simulink model "Final_System_Model_V2"  (R2018a)
settings: Solver=VariableStepAuto  StartTime=0  StopTime=inf  RelTol=1e-3
PreLoadFcn:
  | Ts_Power=1e-6;
  | Ts_Control=100e-6;
undefined symbols (not defined in the file): DiscIntNeverNeededParam, FC, FuelCellLoadFcn, gcbh, Ion, Lithium, sigbuilder_block, sps_rtmsupport
libraries: powerlib x20, simulink x10, fl_lib x8, nesl_utility x6, powerlib_meascontrol x5, electricdrivelib x1, spsFuelCellModel x1, re_lib x1
(part 3 of 4)

== system Final_System_Model_V2/180KW Fuel Cell Stack/Load ==
  note: This Block models the Load Profile as dictated by the ship Resistance in the River Nile
  Signal : Inport
  Bus Selector : BusSelector  OutputSignals=Cell Output Voltage (V),Number Of Cells
  Current from Load profile of one day : Subsystem  Tag=STV Subsys  LoadFcn=sigbuilder_block('load');  StartFcn=sigbuilder_block('start');  StopFcn=sigbuilder_block('stop');  ClipboardFcn=sigbuilder_block('clipboard');  mask(Sigbuilder block){tuvar=[0:10]}
      mask help: Simulink:masks:SigbuilderBlock_MD
      mask init:
      | if ~strcmp(get_param(bdroot(gcbh),'SimulationStatus'),'stopped') tuvar = sigbuilder_block('maskInit'); end
      settings: CopyFcn=sigbuilder_block('copy');  DeleteFcn=sigbuilder_block('delete');  ModelCloseFcn=sigbuilder_block('modelClose');  PreSaveFcn=sigbuilder_block('preSave');  PauseFcn=sigbuilder_block('pause');  ContinueFcn=sigbuilder_block('continue');  NameChangeFcn=sigbuilder_block('namechange');  OpenFcn=sigbuilder_block('open',[403.5 117 550.5 359.25 ]);  CloseFcn=sigbuilder_block('close');
      mask Display: plot(0, 0, 100, 100,[2, 2, 32, 32, 2], [68, 8, 8, 68, 68],[32, 2], [38, 38], [32, 19, 2],[53, 60, 44], [32, 17, 17, 2],[16, 16, 31, 31]);txt = getActiveGroup(gcbh);text(2, 100, txt,'verticalAlignment', 'top');
  Product : Product
  Terminator : Terminator
  Terminator1 : Terminator
  Total Output Voltage (V) : Outport
  wires:
  Signal/1 -> Bus Selector/1
  Bus Selector/1 -> Product/1  "<Cell Output Voltage (V)>"
  Product/1 -> Total Output Voltage (V)/1  "Total Output Voltage (V)"
  Current from Load profile of one day/2(Signal 2) -> Terminator1/1  "Current from Load profile (Alex to Aswan)"
  Bus Selector/2 -> Product/2  "<Number Of Cells>"
  Current from Load profile of one day/1(Signal 1) -> Terminator/1  "Current from Load profile (Alex to Aswan)"

== system Final_System_Model_V2/DC-DC converter/Subsystem ==
  duty cycle : Inport
  I in : Inport  Port=2
  V in : Inport  Port=3
  Constant : Constant
  I out : Product  Inputs=*/
  Multiply : Product
  Multiply1 : Product
  Subtract : Sum  Inputs=+-
  V out : Product  Inputs=*/
  efficiency : Gain  Gain=0.98
  efficiency1 : Gain  Gain=0.98
  I o : Outport
  V o : Outport  Port=2
  wires:
  Subtract/1 -> Multiply/1, V out/2
  efficiency/1 -> Multiply/2
  Multiply/1 -> I out/1
  Constant/1 -> Subtract/1
  duty cycle/1 -> Subtract/2, I out/2, Multiply1/2
  Multiply1/1 -> V out/1
  efficiency1/1 -> Multiply1/1
  I in/1 -> efficiency/1
  V out/1 -> V o/1
  I out/1 -> I o/1
  V in/1 -> efficiency1/1

== system Final_System_Model_V2/DC-DC converter/duty cycle ==
  V in : Inport
  V req : Inport  Port=2
  Add : Sum
  Constant : Constant
  Divide : Product  Inputs=*/
  Gain : Gain  Gain=0.98
  Subtract : Sum  Inputs=+-
  tag scope: duty_cycle=global
  wires:
  Subtract/1 -> [duty_cycle]
  V req/1 -> Add/2
  V in/1 -> Gain/1
  Constant/1 -> Subtract/1
  Add/1 -> Divide/2
  Gain/1 -> Divide/1, Add/1
  Divide/1 -> Subtract/2

== system Final_System_Model_V2/Electrolyzer Stack/electrolyser stack ==
  In1 : Inport
  In2 : Inport  Port=2
  Gain : Gain  Gain=2
  Multiply : Product
  Multiply1 : Product
  area in cm^2 : Constant  Value=428
  electrolyser cell : Subsystem
  number of cells : Constant  Value=212
  voltage : Scope
  Out1 : Outport
  Out3 : Outport  Port=2
  wires:
  area in cm^2/1 -> electrolyser cell/3(In3)
  Multiply/1 -> Out1/1
  number of cells/1 -> Multiply1/1, Multiply/1
  electrolyser cell/1(Out1) -> voltage/1, Multiply/2
  In1/1 -> electrolyser cell/1(In1)
  In2/1 -> electrolyser cell/2(In2)
  electrolyser cell/2(Out2) -> Gain/1
  Gain/1 -> Multiply1/2
  Multiply1/1 -> Out3/1

== system Final_System_Model_V2/OLD Version Models/Electrolyser ==
  In1 : Inport
  Electrolyser : Subsystem
  Kg/h : Outport
  wires:
  Electrolyser/1(Kg/h) -> Kg/h/1
  In1/1 -> Electrolyser/1(Current (A))

== system Final_System_Model_V2/OLD Version Models/Fuel Cell ==
  "Hydrogen Flow Rate (kg/s) " : Inport
  Fuel Mass Flow Rate (kg/s) To Current (A) : Subsystem
  Gain : Gain  Gain=0.001
  Number of Cells : Constant  Value=208
  Product : Product
  Output Current : Outport
  Output Voltage (V) : Outport  Port=2
  Output Power (KW) : Outport  Port=3
  wires:
  Number of Cells/1 -> Fuel Mass Flow Rate (kg/s) To Current (A)/2(Number Of Cells)
  "Hydrogen Flow Rate (kg/s) "/1 -> Fuel Mass Flow Rate (kg/s) To Current (A)/1(Hydrogen Flow Rate (kg/s))
  Fuel Mass Flow Rate (kg/s) To Current (A)/1(Current (A)) -> Product/1, Output Current/1
  Fuel Mass Flow Rate (kg/s) To Current (A)/2(Output Voltage (V)) -> Product/2, Output Voltage (V)/1
  Product/1 -> Gain/1
  Gain/1 -> Output Power (KW)/1

== system Final_System_Model_V2/OLD Version Models/Fuel Cell Stack ==
  FuelFr : Inport
  AirFr : Constant  Value=FC.Uf_O2
  Controlled Voltage Source1 : powerlib/Electrical Sources/Controlled Voltage Source  Initialize=on  Source_Type=AC  Amplitude=0  Phase=0  Frequency=0  Measurements=None
  Current Measurement1 : powerlib/Measurements/Current Measurement  PhasorSimulation=off  OutputType=Complex  PSBequivalent=0
  Diode1 : powerlib/Power Electronics/Diode  Ron=FC.Rohm  Lon=0  Vf=0  IC=0  UseSnubber=off  Rs=1e4  Cs=inf  Measurements=off
  Gain1 : Gain  Gain=0.01
  Gain3 : Gain  Gain=0.01
  Model : Subsystem  BlockChoice=Discrete/Detailed
      settings: AttributesFormatString=%<BlockChoice>  TemplateBlock=spsFuelCellModel/Fuel Cell model  MemberBlocks=Continuous/Detailed,Continuous/Simplified,Discrete/Detailed,Discrete/Simplified
  PAir : Constant  Value=FC.PAir
  Pfuel : Constant  Value=FC.Pf
  T : Constant  Value=FC.Tnom
  x_H2 : Constant  Value=FC.x*100
  y_O2 : Constant  Value=FC.y*100
  + : PMIOPort  Tag=PMCPort  Side=Right
  - : PMIOPort  Tag=PMCPort  Port=2  Side=Right
  m : Outport
  wires:
  PAir/1 -> Model/8(PAir)
  Pfuel/1 -> Model/7(Pf)
  T/1 -> Model/2(Op Temp)
  Model/1(Voltage) -> Controlled Voltage Source1/1
  Current Measurement1/1 -> Model/1(Current)
  Model/2(m) -> m/1
  FuelFr/1 -> Model/3(H2)
  x_H2/1 -> Gain1/1
  AirFr/1 -> Model/5(Air)
  y_O2/1 -> Gain3/1
  Gain1/1 -> Model/4(x_H2)
  Gain3/1 -> Model/6(y_O2)
  connections:
  Current Measurement1/LConn1 -- Controlled Voltage Source1/RConn1
  Current Measurement1/RConn1 -- Diode1/LConn1
  -/RConn1 -- Controlled Voltage Source1/LConn1
  Diode1/RConn1 -- +/RConn1

== system Final_System_Model_V2/OLD Version Models/Subsystem ==
  duty_cycle : Inport
  I in : Inport  Port=2
  V in : Inport  Port=3
  Constant : Constant
  I out : Product  Inputs=*/
  Multiply : Product
  Multiply1 : Product
  Subtract : Sum  Inputs=+-
  V out : Product  Inputs=*/
  efficiency : Gain  Gain=0.98
  efficiency1 : Gain  Gain=0.98
  I o : Outport
  V o : Outport  Port=2
  wires:
  Subtract/1 -> Multiply/1, V out/2
  efficiency/1 -> Multiply/2
  Multiply/1 -> I out/1
  Constant/1 -> Subtract/1
  duty_cycle/1 -> Subtract/2, I out/2, Multiply1/2
  Multiply1/1 -> V out/1
  efficiency1/1 -> Multiply1/1
  I in/1 -> efficiency/1
  V out/1 -> V o/1
  I out/1 -> I o/1
  V in/1 -> efficiency1/1

== system Final_System_Model_V2/OLD Version Models/TANK ==
  Input Hydrogen From Electrolyzer (Kg/s) : Inport
  Clock : Clock
  Constant : Constant  Value=700
  Divide : Product  Inputs=*/
  If : If  IfExpression=u1 >= 70.91e6  ShowElse=off
  If Action Subsystem : Subsystem  TreatAsAtomicUnit=on
  J/kgK : Constant  Value=4124.3
  Product : Product
  Product1 : Product  Inputs=3
  Saturation : Saturate  UpperLimit=700  LowerLimit=1
  Simulink-PS Converter : nesl_utility/Simulink-PS Converter  PhysicalDomain=network_engine_domain  SubClassName=ps_input  LeftPortType=input  RightPortType=output  PseudoPeriodic=off  Frequencies=[]  NoiseDistribution=none  NoiseParameters=[]  Unit=Pa  AffineConversion=off  FilteringAndDerivatives=provide  SimscapeFilterOrder=1  InputFilterTimeConstant=0.001  UdotUserProvided=0
  Simulink-PS Converter1 : nesl_utility/Simulink-PS Converter  PhysicalDomain=network_engine_domain  SubClassName=ps_input  LeftPortType=input  RightPortType=output  PseudoPeriodic=off  Frequencies=[]  NoiseDistribution=none  NoiseParameters=[]  Unit=K  AffineConversion=off  FilteringAndDerivatives=provide  SimscapeFilterOrder=1  InputFilterTimeConstant=0.001  UdotUserProvided=0
  Tank Volume (m^3) : Constant
  Temp (K) : Constant  Value=353.15
  Pressure (Pa) : PMIOPort  Side=Right
  Temp1 (K) : PMIOPort  Port=2  Side=Right
  wires:
  Product1/1 -> Divide/1
  Temp (K)/1 -> Simulink-PS Converter1/1, Product1/3
  Input Hydrogen From Electrolyzer (Kg/s)/1 -> Product/1
  Tank Volume (m^3)/1 -> Divide/2
  If Action Subsystem/1(Out1) -> Saturation/1
  Clock/1 -> Product/2
  If/1 -> If Action Subsystem/Action
  Product/1 -> Product1/1  "Mass in Tank (Kg)"
  Divide/1 -> If/1  "Pressure (Pa)"
  Constant/1 -> If Action Subsystem/1(In1)
  J/kgK/1 -> Product1/2
  Saturation/1 -> Simulink-PS Converter/1
  connections:
  Pressure (Pa)/RConn1 -- Simulink-PS Converter/RConn1
  Temp1 (K)/RConn1 -- Simulink-PS Converter1/RConn1

== system Final_System_Model_V2/OLD Version Models/converter ==
  In1 : Inport
  In2 : Inport  Port=2
  Divide : Product  Inputs=*/
  Gain : Gain  Gain=0.98
  Out1 : Outport
  wires:
  Gain/1 -> Divide/2
  In1/1 -> Divide/1
  Divide/1 -> Out1/1
  In2/1 -> Gain/1

== system Final_System_Model_V2/Solar Panel + Solar Charge Controller/PV Insert inputs here ==
  V_PV : Inport
  PV num : Inport  Port=2
  I_sc : Constant  Value=6.39
  Ns_cells : Constant  Value=96
  Product : Product
  Rp : Constant  Value=884.5
  Scope : Scope
  Subsystem : Subsystem
  Temp : Step  Time=5  Before=25  After=25  SampleTime=0
  V_oc : Constant  Value=68.2
  radiation ratio : Step  Before=1  SampleTime=0
  I_PV : Outport
  wires:
  Subsystem/1(I_PV) -> Scope/1, Product/2  "I_PV(A)"
  Temp/1 -> Subsystem/3(T_o)  "Temperature(c)"
  radiation ratio/1 -> Subsystem/2(insolation)  "Radiation ratio"
  Rp/1 -> Subsystem/4(Rp)  "Rp(ohm)"
  V_PV/1 -> Subsystem/1(V_PV)  "V_PV (volt)"
  Product/1 -> I_PV/1
  PV num/1 -> Product/1
  I_sc/1 -> Subsystem/5(I_sc)
  Ns_cells/1 -> Subsystem/6(Ns cells)
  V_oc/1 -> Subsystem/7(V_oc)

== system Final_System_Model_V2/Solar Panel + Solar Charge Controller/Solar Charge Controller ==
  note: 5 kHz - 500V
      | Boost Converter
  m : Inport
  Bus Selector : BusSelector  OutputSignals=V_PV,I_PV
  C1 : powerlib/Elements/Series RLC Branch  LConnTagsString=__new0  RConnTagsString=__new0  BranchType=C  Resistance=1.0  Inductance=1.0  SetiL0=off  InitialCurrent=0  Capacitance=12000e-06  Setx0=off  InitialVoltage=0  Measurements=None
  C2 : powerlib/Elements/Series RLC Branch  LConnTagsString=__new0  RConnTagsString=__new0  BranchType=C  Resistance=1.0  Inductance=1.0  SetiL0=off  InitialCurrent=0  Capacitance=12000e-06  Setx0=off  InitialVoltage=0  Measurements=None
  C3 : powerlib/Elements/Series RLC Branch  LConnTagsString=__new0  RConnTagsString=__new0  BranchType=C  Resistance=1.0  Inductance=1.0  SetiL0=off  InitialCurrent=0  Capacitance=100e-6  Setx0=off  InitialVoltage=0  Measurements=Branch voltage
  Deblock Converters : Step  Time=.05  SampleTime=0
  Diode1 : powerlib/Power Electronics/Diode  Ron=1e-4  Lon=0  Vf=0  IC=0  UseSnubber=off  Rs=inf  Cs=inf  Measurements=off
  IGBT1 : powerlib/Power Electronics/IGBT  Ron=0.001  Lon=0  Vf=0  Tf=0  Tt=0  IC=0  Rs=1e5  Cs=inf  Measurements=off
  L1 : powerlib/Elements/Series RLC Branch  LConnTagsString=__new0  RConnTagsString=__new0  BranchType=RL  Resistance=0.005  Inductance=5e-3  SetiL0=off  InitialCurrent=0  Capacitance=1e-6  Setx0=off  InitialVoltage=0  Measurements=None
  "MPPT Controller using  \"Incremental Conductance + Integral Regulator \"  technique " : Subsystem  mask(Boost Control - MPPT){fc=5000, T_MPPT=200e-6, Dinit=0.5}
      mask prompts: fc "PWM switching frequency (Hz)"; T_MPPT "Time window used by MPPT control (s)"; Dinit "Initial value of duty cycle"
  Product : Product
  Product2 : Product  RndMeth=Zero
  "+ " : PMIOPort  Side=Left
  - : PMIOPort  Port=2  Side=Left
  Voltage : Outport
  Current : Outport  Port=2
  Power : Outport  Port=3
  wires:
  Product2/1 -> IGBT1/1
  "MPPT Controller using  \"Incremental Conductance + Integral Regulator \"  technique "/1(Pulses) -> Product2/2
  Deblock Converters/1 -> Product2/1
  Bus Selector/2 -> Product/2, Current/1, "MPPT Controller using  \"Incremental Conductance + Integral Regulator \"  technique "/2(I_PV)  "<I_PV>"
  Bus Selector/1 -> Product/1, Voltage/1, "MPPT Controller using  \"Incremental Conductance + Integral Regulator \"  technique "/1(V_PV)  "<V_PV>"
  m/1 -> Bus Selector/1
  Product/1 -> Power/1
  connections:
  C2/LConn1 -- C1/RConn1
  C3/LConn1 -- "+ "/RConn1 -- L1/LConn1
  C1/LConn1 -- Diode1/RConn1
  L1/RConn1 -- Diode1/LConn1 -- IGBT1/LConn1
  C2/RConn1 -- IGBT1/RConn1 -- C3/RConn1 -- -/RConn1

== system Final_System_Model_V2/Solar Panel + Solar Charge Controller/Solar Charge Controller MPPT it is a device which track a point which has the max power ==
  I'_PV : Inport
  PV num : Inport  Port=2
  Divide : Product  Inputs=*/
  "MPPT " : Subsystem
  I_PV : Outport
  "V'_PV " : Outport  Port=2
  wires:
  "MPPT "/1(V_mpp) -> "V'_PV "/1, "MPPT "/2(V_PV)  "V_PV(Volt)"
  I'_PV/1 -> I_PV/1, Divide/1
  Divide/1 -> "MPPT "/1(I_PV)
  PV num/1 -> Divide/2

== system Final_System_Model_V2/Tank/Subsystem ==
  Reset Order : Inport
  Add1 : Sum  Inputs=+-
  Clock2 : Clock
  Clock3 : Clock
  Constant5 : Constant  Value=0
  Constant6 : Constant
  Gain : Gain  Gain=-1
  If : If  ShowElse=off
  If Action Subsystem : Subsystem  TreatAsAtomicUnit=on
  Pulse Generator : DiscretePulseGenerator  PulseType=Time based  TimeSource=Use external signal  Period=0.1  PulseWidth=5
  Scope : Scope
  Switch3 : Switch  Criteria=u2 > Threshold
  Clock100 : Outport
  wires:
  Pulse Generator/1 -> Switch3/1
  Gain/1 -> Clock100/1, Scope/1
  Add1/1 -> Gain/1
  Constant6/1 -> Pulse Generator/1
  If/1 -> If Action Subsystem/Action
  Switch3/1 -> If/1
  If Action Subsystem/1(Out1) -> Add1/1
  Clock2/1 -> Add1/2
  Constant5/1 -> Switch3/3
  Clock3/1 -> If Action Subsystem/1(In1)
  Reset Order/1 -> Switch3/2

== system Final_System_Model_V2/Tank/Subsystem1 ==
  Reset Order : Inport
  Add1 : Sum  Inputs=+-
  Clock2 : Clock
  Clock3 : Clock
  Constant5 : Constant  Value=0
  Constant6 : Constant
  Gain : Gain  Gain=-1
  If : If  ShowElse=off
  If Action Subsystem : Subsystem  TreatAsAtomicUnit=on
  Pulse Generator : DiscretePulseGenerator  PulseType=Time based  TimeSource=Use external signal  Period=0.1  PulseWidth=5
  Scope : Scope
  Switch3 : Switch  Criteria=u2 > Threshold
  Clock100 : Outport
  wires:
  Pulse Generator/1 -> Switch3/1
  Gain/1 -> Clock100/1, Scope/1
  Add1/1 -> Gain/1
  Constant6/1 -> Pulse Generator/1
  If/1 -> If Action Subsystem/Action
  Switch3/1 -> If/1
  If Action Subsystem/1(Out1) -> Add1/1
  Clock2/1 -> Add1/2
  Constant5/1 -> Switch3/3
  Clock3/1 -> If Action Subsystem/1(In1)
  Reset Order/1 -> Switch3/2

== system Final_System_Model_V2/Tank Control/trigger Pulse ==
  Trigger : Inport
  Scope : Scope
  Subsystem : Subsystem
  pert magnitude : Constant
  pert magnitude1 : Constant  Value=0.4
  Reset Charge Clock output : Outport
  wires:
  Trigger/1 -> Subsystem/3(Activation (0 or 1))
  Subsystem/1(Pulse) -> Reset Charge Clock output/1, Scope/1
  pert magnitude1/1 -> Subsystem/1(Pulse Width (sec))
  pert magnitude/1 -> Subsystem/2(Pulse Amplitude)

== system Final_System_Model_V2/Tank Control/trigger Pulse1 ==
  Trigger : Inport
  Scope : Scope
  Subsystem : Subsystem
  pert magnitude : Constant
  pert magnitude1 : Constant  Value=0.4
  Reset Discharge Clock output : Outport
  wires:
  pert magnitude/1 -> Subsystem/2(Pulse Amplitude)
  pert magnitude1/1 -> Subsystem/1(Pulse Width (sec))
  Subsystem/1(Pulse) -> Scope/1, Reset Discharge Clock output/1
  Trigger/1 -> Subsystem/3(Activation (0 or 1))

== system Final_System_Model_V2/180KW Fuel Cell Stack/From Load Current and Fuel Cell Output Current (A) to Valve Restriction Area (m^2)/Subsystem ==
  In1 : Inport
  Add1 : Sum  Inputs=4
  Bus Creator1 : BusCreator  Inputs=7
  Bus Selector1 : BusSelector  OutputSignals=Output Current (A),3,3:0735e-14,Output Current (A),2,-5:0428e-11,Output Current (A),4:1772e-08,2:7105e-07
  Constant10 : Constant  Value=4.1772e-08
  Constant11 : Constant  Value=2.7105e-07
  Constant6 : Constant  Value=3
  Constant7 : Constant  Value=3.0735e-14
  Constant8 : Constant  Value=2
  Constant9 : Constant  Value=-5.0428e-11
  Math Function2 : Math  Operator=pow  SaturateOnIntegerOverflow=on
  Math Function3 : Math  Operator=pow  SaturateOnIntegerOverflow=on
  Product3 : Product
  Product4 : Product
  Product5 : Product
  Unit Delay3 : UnitDelay  SampleTime=-1
  Valve Opening from Output Current : Outport
  wires:
  Product3/1 -> Add1/1
  Constant9/1 -> Bus Creator1/5  "-5:0428e-11"
  Constant11/1 -> Bus Creator1/7  "2:7105e-07"
  Constant8/1 -> Bus Creator1/4  "2"
  Constant6/1 -> Bus Creator1/2  "3"
  Bus Selector1/5 -> Math Function3/2  "<2>"
  Constant10/1 -> Bus Creator1/6  "4:1772e-08"
  In1/1 -> Unit Delay3/1
  Math Function2/1 -> Product3/1
  Math Function3/1 -> Product4/1
  Bus Selector1/3 -> Product3/2  "<3:0735e-14>"
  Bus Selector1/9 -> Add1/4  "<2:7105e-07>"
  Bus Selector1/2 -> Math Function2/2  "<3>"
  Bus Creator1/1 -> Bus Selector1/1
  Bus Selector1/6 -> Product4/2  "<-5:0428e-11>"
  Bus Selector1/8 -> Product5/2  "<4:1772e-08>"
  Bus Selector1/4 -> Math Function3/1  "<Output Current (A)>"
  Product4/1 -> Add1/2
  Product5/1 -> Add1/3
  Constant7/1 -> Bus Creator1/3  "3:0735e-14"
  Unit Delay3/1 -> Bus Creator1/1  "Output Current (A)"
  Bus Selector1/7 -> Product5/1  "<Output Current (A)>"
  Bus Selector1/1 -> Math Function2/1  "<Output Current (A)>"
  Add1/1 -> Valve Opening from Output Current/1  "Valve Opening from Output Current"

== system Final_System_Model_V2/180KW Fuel Cell Stack/From Load Current and Fuel Cell Output Current (A) to Valve Restriction Area (m^2)/Subsystem1 ==
  In1 : Inport
  Add : Sum  Inputs=4
  Bus Creator : BusCreator  Inputs=7
  Bus Selector : BusSelector  OutputSignals=|
      | Load Profile Current (A).Required Current
      | (A),3,3:0735e-14,Load Profile Current (A).Required Current
      | (A),2,-5:0428e-11,Load Profile Current (A).Required Current
      | (A),4:1772e-08,2:7105e-07
  Constant : Constant  Value=3
  Constant1 : Constant  Value=3.0735e-14
  Constant2 : Constant  Value=2
  Constant3 : Constant  Value=-5.0428e-11
  Constant4 : Constant  Value=4.1772e-08
  Constant5 : Constant  Value=2.7105e-07
  Math Function : Math  Operator=pow  SaturateOnIntegerOverflow=on
  Math Function1 : Math  Operator=pow  SaturateOnIntegerOverflow=on
  Product : Product
  Product1 : Product
  Product2 : Product
  Unit Delay2 : UnitDelay  SampleTime=-1
  Out1 : Outport
  wires:
  Bus Selector/2 -> Math Function/2  "<3>"
  Bus Selector/5 -> Math Function1/2  "<2>"
  Product/1 -> Add/1
  Constant/1 -> Bus Creator/2  "3"
  Unit Delay2/1 -> Bus Creator/1  "Load Profile Current (A)"
  Constant5/1 -> Bus Creator/7  "2:7105e-07"
  Constant2/1 -> Bus Creator/4  "2"
  Bus Selector/1 -> Math Function/1  "<Required Current (A)>"
  Constant3/1 -> Bus Creator/5  "-5:0428e-11"
  Constant4/1 -> Bus Creator/6  "4:1772e-08"
  Bus Selector/7 -> Product2/1  "<Required Current (A)>"
  Math Function1/1 -> Product1/1
  Bus Selector/9 -> Add/4  "<2:7105e-07>"
  Bus Selector/8 -> Product2/2  "<4:1772e-08>"
  Bus Selector/6 -> Product1/2  "<-5:0428e-11>"
  Constant1/1 -> Bus Creator/3  "3:0735e-14"
  Product1/1 -> Add/2
  Math Function/1 -> Product/1
  Bus Creator/1 -> Bus Selector/1
  Product2/1 -> Add/3
  Bus Selector/3 -> Product/2  "<3:0735e-14>"
  Bus Selector/4 -> Math Function1/1  "<Required Current (A)>"
  In1/1 -> Unit Delay2/1
  Add/1 -> Out1/1

== system Final_System_Model_V2/180KW Fuel Cell Stack/Fuel Cell Model/ From Current Density (A//cm^2) To Overvoltages (V) ==
  note: This Block calculates all the Resistances in the Fuel Cell
      | 1-Activation Overvoltage 2- Ohmic Overvoltage 3-Concentration Overvoltage
      | INPUTS: INPUTS: A) Current Density (A/cm^2) INPUTS: A) Current Density (A/cm^2)
      | A) Current Density (A/cm^2) OUTPUTS: A) Ohmic Overvoltage (V) OUTPUTS: A) Concentration Overvoltage (V)
      | B) Temperature (c)
      |
      | OUTPUTS:
      | A) Activation Overvoltage (V)
  Current Density (A/cm^2) : Inport
  Temperature (C) : Inport  Port=2
  Activation Overvoltage : Subsystem
  Concentration Overvoltage : Subsystem
  Ohmic Overvoltage : Subsystem
  Activation Overvoltage (V) : Outport
  Ohmic Overvoltage (V) : Outport  Port=2
  Concentration Overvoltage (V) : Outport  Port=3
  Exchange Current Density (i_0) : Outport  Port=4
  wires:
  Temperature (C)/1 -> Activation Overvoltage/1(Temperature/C1)
  Current Density (A/cm^2)/1 -> Activation Overvoltage/2(Current Density (i)(A/cm^2)), Concentration Overvoltage/1(Current Density (i)1), Ohmic Overvoltage/1(Current Density (i ))
  Ohmic Overvoltage/1(V_Resistive) -> Ohmic Overvoltage (V)/1
  Activation Overvoltage/1(Activation Overvoltage1 (V)) -> Activation Overvoltage (V)/1
  Concentration Overvoltage/1("Concentration Overvoltage1 (V) ") -> Concentration Overvoltage (V)/1
  Activation Overvoltage/2(Exchange Current Density (i_0)) -> Exchange Current Density (i_0)/1

== system Final_System_Model_V2/180KW Fuel Cell Stack/Fuel Cell Model/Air Flow Rate To Current (A) ==
  note: The function of this block is: To calculate the Air Mass Flow Rate in (kg/s) using the Input Current Density (A/cm^2)
      | Inputs: Outputs:
      | a) Current DEnsity (A/cm^2) A) Air Mass Flow Rate (kg/s)
      | b) Cell Area (cm^2)
      | c) Number of Cells
  Current Density (A/cm^2) : Inport
  Cell Area (cm^2) : Inport  Port=2
  Number Of Cells : Inport  Port=3
  Air Molar Mass (Kg) : Constant  Value=28.9647e-3
  Current (A) : Product
  Divide : Product  Inputs=*/
  From Stack Current (A) To Oxygen Mass Flow Rate(kg/s) : Subsystem
  Oxygen Molar Mass per One Mole of Air (Kg) : Constant  Value=6.72e-3
  Product : Product
  Air Mass Flow Rate (kg/s) : Outport
  wires:
  Current (A)/1 -> From Stack Current (A) To Oxygen Mass Flow Rate(kg/s)/1(Current (A))
  Number Of Cells/1 -> From Stack Current (A) To Oxygen Mass Flow Rate(kg/s)/2(Number Of Cells)
  From Stack Current (A) To Oxygen Mass Flow Rate(kg/s)/1(Oxygen Flow Rate (kg/s)) -> Product/1
  Current Density (A/cm^2)/1 -> Current (A)/1
  Cell Area (cm^2)/1 -> Current (A)/2
  Air Molar Mass (Kg)/1 -> Product/2
  Product/1 -> Divide/1
  Oxygen Molar Mass per One Mole of Air (Kg)/1 -> Divide/2
  Divide/1 -> Air Mass Flow Rate (kg/s)/1  "Air Mass Flow Rate (kg/s)"

== system Final_System_Model_V2/180KW Fuel Cell Stack/Fuel Cell Model/Current Density A//cm^2 (Polarization Curve) ==
  Demux : Demux  Tag=STV Demux  Outputs=2
  FromWs : FromWorkspace  Tag=STV FromWs  VariableName=tuvar  SampleTime=0
      SigBuilderData=|
      | common.afterFinalStr = 'Extrapolate'
      | common.sampleTime = 0
      | dataSet.timeRange = [0 20]
      | dataSet.name = 'Group 1'
      | sbobj.Groups.Name = 'Group 1'
      | sbobj.Groups.Signals(1).Name = 'Signal 1'
      | sbobj.Groups.Signals(1).XData = [0 0.5 1 20]
      | sbobj.Groups.Signals(1).YData = [0.01 1 1.4 1.4]
      | sbobj.Groups.Signals(2).Name = 'Signal 2'
      | sbobj.Groups.Signals(2).XData = [0 20]
      | sbobj.Groups.Signals(2).YData = [1 1]
      | sbobj.Groups.TimeRange = [0 20]
  Signal 1 : Outport  Tag=STV Outport
  Signal 2 : Outport  Tag=STV Outport  Port=2
  wires:
  Demux/1 -> Signal 1/1
  FromWs/1 -> Demux/1
  Demux/2 -> Signal 2/1

== system Final_System_Model_V2/180KW Fuel Cell Stack/Fuel Cell Model/From Mass Flow Rates (kg//s) To Current Density (A//cm^2) ==
  note: The function of this block is to convert the input Hydrogen Mass Flow rate (Kg/s) to Current (A) then divide it by the Cell Area (cm^2) to get (Current Density) (A/cm^2)
      | which will be the input of several other blocks.
      | Inputs: a)Hydrogen Mass Flow Rate (kg/s) Outputs: Current Density (A/cm^2)
      | b)Number of Cells
      | c) Cell Area (cm^2)
  Hydrogen Flow Rate (kg/s) : Inport
  Cell Area (cm^2) : Inport  Port=2
  Number Of Cells : Inport  Port=3
  From Current (A) To Current Density (A/cm^2) : Subsystem
  Fuel Mass Flow Rate (kg/s) To Current (A) : Subsystem
  Current Density (A/cm^2) : Outport
  wires:
  Cell Area (cm^2)/1 -> From Current (A) To Current Density (A/cm^2)/2(Cell Area (cm^2))
  Fuel Mass Flow Rate (kg/s) To Current (A)/1(Current (A)) -> From Current (A) To Current Density (A/cm^2)/1(Nominal Current (A))
  Hydrogen Flow Rate (kg/s)/1 -> Fuel Mass Flow Rate (kg/s) To Current (A)/1(Hydrogen Flow Rate (kg/s))
  From Current (A) To Current Density (A/cm^2)/1(Current Density (A/cm^2)) -> Current Density (A/cm^2)/1  "Current density (A/cm^2)"
  Number Of Cells/1 -> Fuel Mass Flow Rate (kg/s) To Current (A)/2(Number Of Cells)  "Number Of Cells"

== system Final_System_Model_V2/180KW Fuel Cell Stack/Fuel Cell Model/From Pressures (atm) To Nernest Voltage (V) ==
  note: This Block calculates the Partial Pressures of Hydrogen and Oxygen (atm) from their pressures (atm) then uses these values to calculate the Nernest Voltage (V)
      |
      | INPUTS: A) Current Density (i) (A/cm^2) OUTPUTS 1: A) Oxygen Partial Pressure (atm) OUTPUTS 2: A) Nernest Voltage (V)
      | B) Absolute Hydrogen Pressure (atm) B) Water Saturation Pressure (atm)
      | C) Absolute Air Pressure (atm) C) Hydrogen Partial Pressure(atm)
      | D) Temperature (c)
  Current Density (i) : Inport
  Hydrogen Pressure (atm) : Inport  Port=2
  Air Pressure (atm) : Inport  Port=3
  Temperature (C) : Inport  Port=4
  From Absolute Pressure (atm) To Partial Pressures (atm) : Subsystem
  From Partial Pressures (atm) To Nernest Voltage (V) : Subsystem
  Oxygen Partial Pressure : Outport
  Nernest Voltage (V) : Outport  Port=2
  Water Pressure : Outport  Port=3
  wires:
  Temperature (C)/1 -> From Partial Pressures (atm) To Nernest Voltage (V)/4(Temperature/C), From Absolute Pressure (atm) To Partial Pressures (atm)/4(Temperature/C)
  From Absolute Pressure (atm) To Partial Pressures (atm)/1(Hydrogen Partial Pressure (pp_H2)) -> From Partial Pressures (atm) To Nernest Voltage (V)/1(Hydrogen Partial Pressure)
  Hydrogen Pressure (atm)/1 -> From Absolute Pressure (atm) To Partial Pressures (atm)/2(Hydrogen Pressure (P_H2))
  From Partial Pressures (atm) To Nernest Voltage (V)/1(Nernest Voltage1) -> Nernest Voltage (V)/1
  From Absolute Pressure (atm) To Partial Pressures (atm)/2(Oxygen Partial Pressure pp_O2) -> Oxygen Partial Pressure/1, From Partial Pressures (atm) To Nernest Voltage (V)/2(Oxygen Partial Pressure)
  From Absolute Pressure (atm) To Partial Pressures (atm)/3(Water Pressure) -> Water Pressure/1, From Partial Pressures (atm) To Nernest Voltage (V)/3(Water Pressure (P_H2O))
  Current Density (i)/1 -> From Absolute Pressure (atm) To Partial Pressures (atm)/1(Current Density (i ))
  Air Pressure (atm)/1 -> From Absolute Pressure (atm) To Partial Pressures (atm)/3(Air Pressure (P_air))

== system Final_System_Model_V2/180KW Fuel Cell Stack/Load/Current from Load profile of one day ==
  Demux : Demux  Tag=STV Demux  Outputs=2
  FromWs : FromWorkspace  Tag=STV FromWs  VariableName=tuvar  SampleTime=0
      SigBuilderData=|
      | common.afterFinalStr = 'Extrapolate'
      | common.sampleTime = 0
      | dataSet.timeRange = [0 300]
      | dataSet.name = 'Group 1'
      | sbobj.Groups.Name = 'Group 1'
      | sbobj.Groups.Signals(1).Name = 'Signal 1'
      | sbobj.Groups.Signals(1).XData = [0 2.75 2.75 5.75 5.75 10.98 10.98 24 24 24.6 24.6 27.61 27.61 30.61 30.61 33.73 33.73 36.73 48 48 52.19 52.19 55.19 55.19 59.38 59.38 62.38 72 72 84 84 96 96 108 108 120 120 132 132 144 144 146.76 146.76 147.76 147.76 156 156 168 168 175.76 175.76 176.76 176.76 180 180 192 192 204 204 216 216 216.76 216.76 217.76 217.76 228 228 240 240 244.83 244.83 300]
      | sbobj.Groups.Signals(1).YData = [145.4545455 145.4545455 0.01 0.01 145.4545455 145.4545455 0.01 0.01 195.4545455 195.4545455 486.3636364 486.3636364 0.01 0.01 404.5454545 404.5454545 0.01 0.01 0.01 486.3636364 486.3636364 0.01 0.01 486.3636364 486.3636364 0.01 0.01 0.01 463.6363636 463.6363636 0.01 0.01 463.6363636 463.6363636 0.01 0.01 463.6363636 463.6363636 0.01 0.01 463.6363636 463.6363636 0.01 0.01 463.6363636 463.6363636 0.01 0.01 463.6363636 463.6363636 0.01 0.01 463.6363636 463.6363636 0.01 0.01 463.6363636 463.6363636 0.01 0.01 463.6363636 463.6363636 0.01 0.01 463.6363636 463.6363636 0.01 0.01 463.6363636 463.6363636 0.01 0.01]
      | sbobj.Groups.Signals(2).Name = 'Signal 2'
      | sbobj.Groups.Signals(2).XData = [0 300]
      | sbobj.Groups.Signals(2).YData = [243 243]
      | sbobj.Groups.TimeRange = [0 300]
  Signal 1 : Outport  Tag=STV Outport
  Signal 2 : Outport  Tag=STV Outport  Port=2
  wires:
  Demux/1 -> Signal 1/1
  FromWs/1 -> Demux/1
  Demux/2 -> Signal 2/1

== system Final_System_Model_V2/Electrolyzer Stack/electrolyser stack/electrolyser cell ==
  In1 : Inport
  In2 : Inport  Port=2
  In3 : Inport  Port=3
  (1/T)/(1/T_ref) : Subsystem
  Constant2 : Constant  Value=1/298
  Eta_B : Subsystem
  F : Constant  Value=96485.33289
  H2 flow rate : Subsystem
  R : Constant  Value=8.314
  Sum : Sum  Inputs=4
  V_0 : Subsystem
  eta_a : Subsystem
  eta_c : Subsystem
  Out1 : Outport
  Out2 : Outport  Port=2
  wires:
  eta_c/1(Out1) -> Sum/4
  In2/1 -> H2 flow rate/1(In1), eta_c/4(In4), eta_a/3(In3), Eta_B/3(In3)
  R/1 -> eta_a/2(In2), eta_a/4(In4), eta_c/2(In2), Eta_B/1(In1)
  In1/1 -> eta_a/5(In5), eta_c/3(In3), Eta_B/2(In2), (1/T)/(1/T_ref)/1(In1), V_0/1(In1)
  (1/T)/(1/T_ref)/1(Out1) -> eta_a/1(In1), eta_c/1(In1)
  eta_a/1(Out1) -> Sum/3
  Constant2/1 -> Eta_B/4(In4), (1/T)/(1/T_ref)/2(In2)
  Eta_B/1(Out1) -> Sum/2
  F/1 -> eta_a/6(In6), eta_c/5(In5), H2 flow rate/2(In2)
  V_0/1(Out1) -> Sum/1
  Sum/1 -> Out1/1
  In3/1 -> H2 flow rate/3(In3)
  H2 flow rate/1(Out1) -> Out2/1

== system Final_System_Model_V2/OLD Version Models/Electrolyser/Electrolyser ==
  Current (A) : Inport
  Constant : Constant  Value=96485.33289
  Divide : Product  Inputs=*/
  Gain : Gain  Gain=0.001*3600
  Gain1 : Gain  Gain=212
  Kg/h : Outport
  wires:
  Constant/1 -> Divide/2
  Divide/1 -> Gain/1
  Current (A)/1 -> Gain1/1
  Gain1/1 -> Divide/1
  Gain/1 -> Kg/h/1

== system Final_System_Model_V2/OLD Version Models/Fuel Cell/Fuel Mass Flow Rate (kg//s) To Current (A) ==
  note: This block calculates the output Current (A) from the Hydrogen Mass Flow Rate (kg/s)
      | I=Hydrogen Mass Flow Rate (kg/s)*2*F/(M_H2*n)
      | where: I=Current (A)
      | F=Faraday Constant=96487 C/mol
      | M_H2=hydrogen molar mass=2.016*10^-3 kg/mol
      | n=Number of Cells
  Hydrogen Flow Rate (kg/s) : Inport
  Number Of Cells : Inport  Port=2
  Cell Output Voltage (V) : Constant  Value=1.06
  Constant1 : Constant  Value=2
  Divide : Product  Inputs=*/
  F : Constant  Value=96487
  Gain : Gain  Gain=1/3600
  Hydrogen Molar Mass : Constant  Value=2.016e-3
  Product{,1..3} (4 alike) : Product
  Current (A) : Outport
  Output Voltage (V) : Outport  Port=2
  wires:
  F/1 -> Product1/2
  Constant1/1 -> Product1/1
  Product1/1 -> Product/2
  Product/1 -> Divide/1
  Hydrogen Molar Mass/1 -> Product2/1
  Number Of Cells/1 -> Product2/2, Product3/1
  Product2/1 -> Divide/2
  Divide/1 -> Current (A)/1
  Hydrogen Flow Rate (kg/s)/1 -> Gain/1
  Product3/1 -> Output Voltage (V)/1
  Cell Output Voltage (V)/1 -> Product3/2
  Gain/1 -> Product/1

== system Final_System_Model_V2/OLD Version Models/Fuel Cell Stack/Model ==
  Current : Inport
  Op Temp : Inport  Port=2
  H2 : Inport  Port=3
  x_H2 : Inport  Port=4
  Air : Inport  Port=5
  y_O2 : Inport  Port=6
  Pf : Inport  Port=7
  PAir : Inport  Port=8
  Discrete/Detailed : spsFuelCellModel/Discrete//Detailed
  Voltage : Outport
  m : Outport  Port=2
  wires:
  Current/1 -> Discrete/Detailed/1
  Op Temp/1 -> Discrete/Detailed/2
  H2/1 -> Discrete/Detailed/3
  x_H2/1 -> Discrete/Detailed/4
  Air/1 -> Discrete/Detailed/5
  y_O2/1 -> Discrete/Detailed/6
  Pf/1 -> Discrete/Detailed/7
  PAir/1 -> Discrete/Detailed/8
  Discrete/Detailed/1 -> Voltage/1
  Discrete/Detailed/2 -> m/1

== system Final_System_Model_V2/OLD Version Models/TANK/If Action Subsystem ==
  In1 : Inport
  Action Port : ActionPort  ActionType=then
  Out1 : Outport
  wires:
  In1/1 -> Out1/1

== system Final_System_Model_V2/Solar Panel + Solar Charge Controller/PV Insert inputs here/Subsystem ==
  V_PV : Inport
  insolation : Inport  Port=2
  T_o : Inport  Port=3
  Rp : Inport  Port=4
  I_sc : Inport  Port=5
  Ns cells : Inport  Port=6
  V_oc : Inport  Port=7
  "C to K Converter " : Subsystem
  I o : Subsystem
  I on : Subsystem
  "I ph due to radiation " : Subsystem
  I pv : Subsystem
  NsAKt Thermal voltafe : Subsystem
  I_PV : Outport
  wires:
  T_o/1 -> "C to K Converter "/1(T_o)
  insolation/1 -> "I ph due to radiation "/1(insolation)
  "C to K Converter "/2(T_rk) -> I o/2(T_rk), "I ph due to radiation "/3(T_rk)  "T_nK"
  I_sc/1 -> "I ph due to radiation "/4(I_scn), I on/2(I_scn)  "I_scn"
  NsAKt Thermal voltafe/1(Ns*a*Kt) -> I pv/4(Ns*A*Kt1)  "const"
  I on/1(I_on) -> I o/3(I_on)  "I_on"
  "C to K Converter "/1(T_ak) -> "I ph due to radiation "/2(T_ak), I on/1(T_ref), I o/1(T_ak), NsAKt Thermal voltafe/1(T_ak T in kelven)  "T_ak"
  "I ph due to radiation "/1(I_photon) -> I pv/2(I_photon)  "I_ph"
  I pv/1(I_PV) -> I_PV/1
  I o/1(I_o) -> I pv/3(I_o)  "I_o"
  V_PV/1 -> I pv/1(V_PV)
  Rp/1 -> I pv/5(Rp Shunt resistance)
  Ns cells/1 -> I on/3(Num series)
  V_oc/1 -> I on/4(V_oc)

== system Final_System_Model_V2/Solar Panel + Solar Charge Controller/Solar Charge Controller/MPPT Controller using  "Incremental Conductance + Integral Regulator "  technique  ==
  V_PV : Inport
  I_PV : Inport  Port=2
  Add : Sum  Inputs=+-
  Deblock MPPT : Step  Time=0.4  SampleTime=0
  Duty Cycle : Constant  Value=Dinit
  MPPT : Subsystem
  PWM Generator (DC-DC) : powerlib_meascontrol/Pulse & Signal Generators/PWM Generator (DC-DC)  Fsw=fc  Ts=Ts_Power
  Saturation : Saturate  UpperLimit=1  LowerLimit=0
  Pulses : Outport
  wires:
  V_PV/1 -> MPPT/1(V_PV)
  I_PV/1 -> MPPT/2(I_PV)
  PWM Generator (DC-DC)/1 -> Pulses/1
  Deblock MPPT/1 -> MPPT/3(on/off)
  Saturation/1 -> PWM Generator (DC-DC)/1
  Add/1 -> Saturation/1  "D"
  MPPT/1(Delta_D) -> Add/2
  Duty Cycle/1 -> Add/1

== system Final_System_Model_V2/Solar Panel + Solar Charge Controller/Solar Charge Controller MPPT it is a device which track a point which has the max power/MPPT  ==
  note: P&O Algorism to track the max power point
  note: DC_DC Buck Boost Conveter
      |
      | to control the output Voltaage
  I_PV : Inport
  V_PV : Inport  Port=2
  Controlled Current Source : powerlib/Electrical Sources/Controlled Current Source  Initialize=on  Source_Type=DC  Amplitude=0  Phase=0  Frequency=0  Measurements=None
  DC Voltage Source : powerlib/Electrical Sources/DC Voltage Source  Amplitude=55  Measurements=None
  Diode : powerlib/Power Electronics/Diode  Ron=0.001  Lon=0  Vf=0.8  IC=0  UseSnubber=off  Rs=500  Cs=250e-9  Measurements=off
  Mosfet : powerlib/Power Electronics/Mosfet  Ron=0.001  Lon=0  Rd=0.01  Vfd=0  IC=0  Rs=1e5  Cs=inf  Measurements=off
  "P&O " : Subsystem
  Series RLC Branch : powerlib/Elements/Series RLC Branch  LConnTagsString=__new0  RConnTagsString=__new0  BranchType=RL  Resistance=.45  Inductance=1e-3  SetiL0=off  InitialCurrent=0  Capacitance=1e-6  Setx0=off  InitialVoltage=0  Measurements=None
  Series RLC Branch1 : powerlib/Elements/Series RLC Branch  LConnTagsString=__new0  RConnTagsString=__new0  BranchType=C  Resistance=1  Inductance=1e-3  SetiL0=off  InitialCurrent=0  Capacitance=2e-3  Setx0=off  InitialVoltage=0  Measurements=None
  Voltage Measurement : powerlib/Measurements/Voltage Measurement  PhasorSimulation=off  OutputType=Complex  PSBequivalent=0
  V_mpp : Outport
  wires:
  Voltage Measurement/1 -> V_mpp/1
  I_PV/1 -> "P&O "/1(I_pv), Controlled Current Source/1
  V_PV/1 -> "P&O "/2(V_PV)
  "P&O "/1(Signal) -> Mosfet/1
  connections:
  Series RLC Branch/RConn1 -- Mosfet/LConn1 -- Diode/LConn1
  Voltage Measurement/LConn1 -- Series RLC Branch/LConn1 -- Series RLC Branch1/LConn1 -- Controlled Current Source/RConn1
  Voltage Measurement/LConn2 -- DC Voltage Source/LConn1 -- Mosfet/RConn1 -- Series RLC Branch1/RConn1 -- Controlled Current Source/LConn1
  DC Voltage Source/RConn1 -- Diode/RConn1

== system Final_System_Model_V2/Tank/Subsystem/If Action Subsystem ==
  In1 : Inport
  Action Port : ActionPort  ActionType=then
  Out1 : Outport
  wires:
  In1/1 -> Out1/1

== system Final_System_Model_V2/Tank/Subsystem1/If Action Subsystem ==
  In1 : Inport
  Action Port : ActionPort  ActionType=then
  Out1 : Outport
  wires:
  In1/1 -> Out1/1

== system Final_System_Model_V2/Tank Control/trigger Pulse/Subsystem ==
  Pulse Width (sec) : Inport
  Pulse Amplitude : Inport  Port=2
  Activation (0 or 1) : Inport  Port=3
  Divide2 : Product  Inputs=**
  Integrator : Integrator  ExternalReset=either
  Scope : Scope
  Scope1 : Scope
  Scope3 : Scope
  Switch : Switch  Criteria=u2 ~= 0  Threshold=1
  Switch1 : Switch  Criteria=u2 ~= 0  Threshold=1
  Y : RelationalOperator  OutDataTypeStr=boolean  RndMeth=Nearest
  baseline : Constant  Value=0
  reach_pert (boolean)3 : Constant  Value=0
  Pulse : Outport
  wires:
  Integrator/1 -> Y/1, Scope/1
  Pulse Width (sec)/1 -> Divide2/1
  Divide2/1 -> Y/2
  Y/1 -> Switch1/2
  baseline/1 -> Switch/3
  Switch/1 -> Switch1/3, Scope1/1, Integrator/1
  Pulse Amplitude/1 -> Switch/1, Divide2/2
  Switch1/1 -> Scope3/1, Pulse/1
  reach_pert (boolean)3/1 -> Switch1/1
  Activation (0 or 1)/1 -> Integrator/2, Switch/2

== system Final_System_Model_V2/Tank Control/trigger Pulse1/Subsystem ==
  Pulse Width (sec) : Inport
  Pulse Amplitude : Inport  Port=2
  Activation (0 or 1) : Inport  Port=3
  Divide2 : Product  Inputs=**
  Integrator : Integrator  ExternalReset=either
  Scope : Scope
  Scope1 : Scope
  Scope3 : Scope
  Switch : Switch  Criteria=u2 ~= 0  Threshold=1
  Switch1 : Switch  Criteria=u2 ~= 0  Threshold=1
  Y : RelationalOperator  OutDataTypeStr=boolean  RndMeth=Nearest
  baseline : Constant  Value=0
  reach_pert (boolean)3 : Constant  Value=0
  Pulse : Outport
  wires:
  Activation (0 or 1)/1 -> Switch/2, Integrator/2
  reach_pert (boolean)3/1 -> Switch1/1
  Switch1/1 -> Pulse/1, Scope3/1
  Pulse Amplitude/1 -> Divide2/2, Switch/1
  Switch/1 -> Integrator/1, Scope1/1, Switch1/3
  baseline/1 -> Switch/3
  Y/1 -> Switch1/2
  Divide2/1 -> Y/2
  Pulse Width (sec)/1 -> Divide2/1
  Integrator/1 -> Scope/1, Y/1

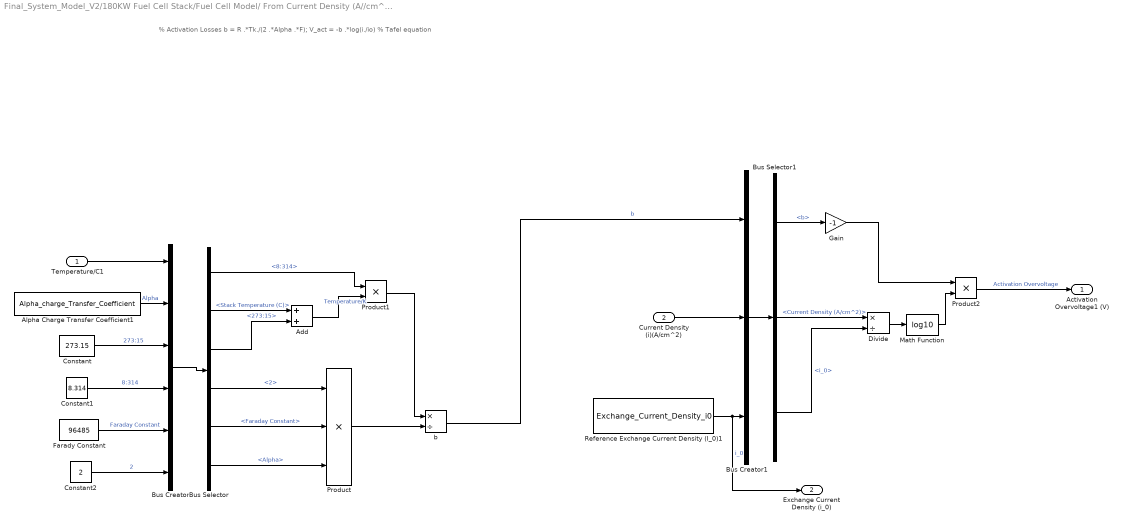
== system Final_System_Model_V2/180KW Fuel Cell Stack/Fuel Cell Model/ From Current Density (A//cm^2) To Overvoltages (V)/Activation Overvoltage ==
  note: % Activation Losses
      | b = R .*Tk./(2 .*Alpha .*F);
      | V_act = -b .*log(i./io) % Tafel equation
  Temperature/C1 : Inport
  Current Density (i)(A/cm^2) : Inport  Port=2
  Add : Sum
  Alpha Charge Transfer Coefficient1 : Constant  Value=Alpha_charge_Transfer_Coefficient
  Bus Creator : BusCreator  Inputs=6
  Bus Creator1 : BusCreator  Inputs=3
  Bus Selector : BusSelector  OutputSignals=8:314,Stack Temperature (C),273:15,2,Faraday Constant,Alpha
  Bus Selector1 : BusSelector  OutputSignals=b,Current Density (A/cm^2),i_0
  Constant : Constant  Value=273.15
  Constant1 : Constant  Value=8.314
  Constant2 : Constant  Value=2
  Divide : Product  Inputs=*/
  Farady Constant : Constant  Value=96485
  Gain : Gain  Gain=-1
  Math Function : Math  Operator=log10  SaturateOnIntegerOverflow=on
  Product : Product  Inputs=3
  Product1 : Product
  Product2 : Product
  Reference Exchange Current Density (I_0)1 : Constant  Value=Exchange_Current_Density_i0
  b : Product  Inputs=*/
  Activation Overvoltage1 (V) : Outport
  Exchange Current Density (i_0) : Outport  Port=2
  wires:
  Alpha Charge Transfer Coefficient1/1 -> Bus Creator/2  "Alpha"
  Temperature/C1/1 -> Bus Creator/1
  Current Density (i)(A/cm^2)/1 -> Bus Creator1/2
  Reference Exchange Current Density (I_0)1/1 -> Bus Creator1/3, Exchange Current Density (i_0)/1  "i_0"
  Product2/1 -> Activation Overvoltage1 (V)/1  "Activation Overvoltage"
  Bus Creator/1 -> Bus Selector/1
  Constant/1 -> Bus Creator/3  "273:15"
  Constant1/1 -> Bus Creator/4  "8:314"
  Farady Constant/1 -> Bus Creator/5  "Faraday Constant"
  Constant2/1 -> Bus Creator/6  "2"
  Bus Selector/4 -> Product/1  "<2>"
  Bus Selector/5 -> Product/2  "<Faraday Constant>"
  Bus Selector/6 -> Product/3  "<Alpha>"
  Product/1 -> b/2
  Bus Selector/1 -> Product1/1  "<8:314>"
  Bus Selector/2 -> Add/1  "<Stack Temperature (C)>"
  Bus Selector/3 -> Add/2  "<273:15>"
  Add/1 -> Product1/2  "Temperature/K"
  Product1/1 -> b/1
  b/1 -> Bus Creator1/1  "b"
  Bus Creator1/1 -> Bus Selector1/1
  Bus Selector1/1 -> Gain/1  "<b>"
  Bus Selector1/2 -> Divide/1  "<Current Density (A/cm^2)>"
  Bus Selector1/3 -> Divide/2  "<i_0>"
  Gain/1 -> Product2/1
  Divide/1 -> Math Function/1
  Math Function/1 -> Product2/2

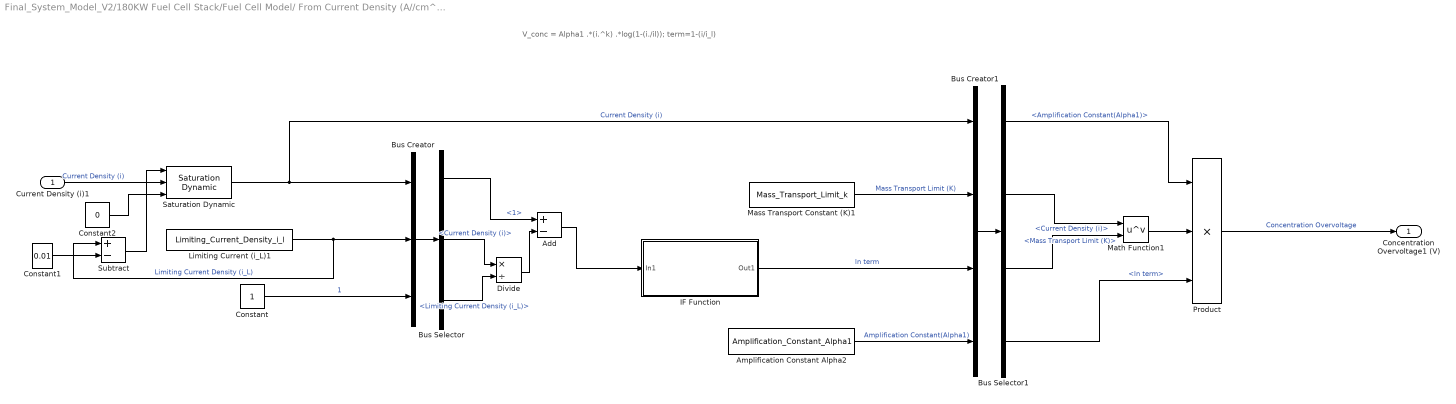
== system Final_System_Model_V2/180KW Fuel Cell Stack/Fuel Cell Model/ From Current Density (A//cm^2) To Overvoltages (V)/Concentration Overvoltage ==
  note: V_conc = Alpha1 .*(i.^k) .*log(1-(i./il));
      | term=1-(i/i_l)
  Current Density (i)1 : Inport
  Add : Sum  Inputs=+-
  Amplification Constant Alpha2 : Constant  Value=Amplification_Constant_Alpha1
  Bus Creator : BusCreator  Inputs=3
  Bus Creator1 : BusCreator  Inputs=4
  Bus Selector : BusSelector  OutputSignals=1,Current Density (i),Limiting Current Density (i_L)
  Bus Selector1 : BusSelector  OutputSignals=Amplification Constant(Alpha1),Current Density (i),Mass Transport Limit (K),ln term
  Constant : Constant
  Constant1 : Constant  Value=0.01
  Constant2 : Constant  Value=0
  Divide : Product  Inputs=*/
  IF Function : Subsystem
  Limiting Current (i_L)1 : Constant  Value=Limiting_Current_Density_i_l
  Mass Transport Constant (K)1 : Constant  Value=Mass_Transport_Limit_k
  Math Function1 : Math  Operator=pow  SaturateOnIntegerOverflow=on
  Product : Product  Inputs=3
  Saturation Dynamic : simulink/Discontinuities/Saturation Dynamic  OutMin=[]  OutMax=[]  OutDataTypeStr=Inherit: Same as second input  OutDataType=fixdt(1, 16)  OutScaling=2^-10  DoSatur=off
  Subtract : Sum  Inputs=+-
  "Concentration Overvoltage1 (V) " : Outport
  wires:
  Bus Creator/1 -> Bus Selector/1
  Limiting Current (i_L)1/1 -> Subtract/1, Bus Creator/2  "Limiting Current Density (i_L)"
  Saturation Dynamic/1 -> Bus Creator1/1, Bus Creator/1  "Current Density (i)"
  Mass Transport Constant (K)1/1 -> Bus Creator1/2  "Mass Transport Limit (K)"
  Amplification Constant Alpha2/1 -> Bus Creator1/4  "Amplification Constant(Alpha1)"
  Product/1 -> "Concentration Overvoltage1 (V) "/1  "Concentration Overvoltage"
  Constant/1 -> Bus Creator/3  "1"
  Bus Selector/1 -> Add/1  "<1>"
  Bus Selector/2 -> Divide/1  "<Current Density (i)>"
  Bus Selector/3 -> Divide/2  "<Limiting Current Density (i_L)>"
  Divide/1 -> Add/2
  Add/1 -> IF Function/1(In1)
  IF Function/1(Out1) -> Bus Creator1/3  "ln term"
  Bus Creator1/1 -> Bus Selector1/1
  Bus Selector1/1 -> Product/1  "<Amplification Constant(Alpha1)>"
  Bus Selector1/2 -> Math Function1/1  "<Current Density (i)>"
  Bus Selector1/3 -> Math Function1/2  "<Mass Transport Limit (K)>"
  Bus Selector1/4 -> Product/3  "<ln term>"
  Math Function1/1 -> Product/2
  Current Density (i)1/1 -> Saturation Dynamic/2  "Current Density (i)"
  Constant1/1 -> Subtract/2
  Subtract/1 -> Saturation Dynamic/1
  Constant2/1 -> Saturation Dynamic/3

== system Final_System_Model_V2/180KW Fuel Cell Stack/Fuel Cell Model/ From Current Density (A//cm^2) To Overvoltages (V)/Ohmic Overvoltage ==
  Current Density (i ) : Inport
  Constant : Constant  Value=-1
  Internal Resistance (r) : Constant  Value=Internal_Resistance_r
  V_Resistive1 : Product  Inputs=3
  V_Resistive : Outport
  wires:
  Constant/1 -> V_Resistive1/3
  Internal Resistance (r)/1 -> V_Resistive1/2
  Current Density (i )/1 -> V_Resistive1/1
  V_Resistive1/1 -> V_Resistive/1  "Ohmic Overvoltage (V)"

== system Final_System_Model_V2/180KW Fuel Cell Stack/Fuel Cell Model/Air Flow Rate To Current (A)/From Stack Current (A) To Oxygen Mass Flow Rate(kg//s) ==
  Current (A) : Inport
  Number Of Cells : Inport  Port=2
  Divide : Product  Inputs=*/
  F : Constant  Value=96487
  Oxygen Molar Mass (Kg/mol) : Constant  Value=32e-3
  Product : Product
  Product1 : Product
  Product2 : Product
  c : Constant  Value=4
  Oxygen Flow Rate (kg/s) : Outport
  wires:
  F/1 -> Product1/1
  Current (A)/1 -> Product/1
  Product/1 -> Divide/1
  Oxygen Molar Mass (Kg/mol)/1 -> Product2/2
  c/1 -> Product1/2
  Divide/1 -> Product2/1
  Product1/1 -> Divide/2
  Product2/1 -> Oxygen Flow Rate (kg/s)/1
  Number Of Cells/1 -> Product/2

== system Final_System_Model_V2/180KW Fuel Cell Stack/Fuel Cell Model/From Mass Flow Rates (kg//s) To Current Density (A//cm^2)/From Current (A) To Current Density (A//cm^2) ==
  note: i=I/A
      | where i=Current Density (A/cm^2)
      | I= Current (A)
      | A=Cell Area (cm^2)
  Nominal Current (A) : Inport
  Cell Area (cm^2) : Inport  Port=2
  Divide : Product  Inputs=*/
  Current Density (A/cm^2) : Outport
  wires:
  Nominal Current (A)/1 -> Divide/1
  Cell Area (cm^2)/1 -> Divide/2
  Divide/1 -> Current Density (A/cm^2)/1

== system Final_System_Model_V2/180KW Fuel Cell Stack/Fuel Cell Model/From Mass Flow Rates (kg//s) To Current Density (A//cm^2)/Fuel Mass Flow Rate (kg//s) To Current (A) ==
  note: This block calculates the output Current (A) from the Hydrogen Mass Flow Rate (kg/s)
      | I=Hydrogen Mass Flow Rate (kg/s)*2*F/(M_H2*n)
      | where: I=Current (A)
      | F=Faraday Constant=96487 C/mol
      | M_H2=hydrogen molar mass=2.016*10^-3 kg/mol
      | n=Number of Cells
  Hydrogen Flow Rate (kg/s) : Inport
  Number Of Cells : Inport  Port=2
  Constant1 : Constant  Value=2
  Divide : Product  Inputs=*/
  F : Constant  Value=96487
  Hydrogen Molar Mass : Constant  Value=2.016e-3
  Product : Product
  Product1 : Product
  Product2 : Product
  Current (A) : Outport
  wires:
  F/1 -> Product1/2
  Constant1/1 -> Product1/1
  Product1/1 -> Product/2
  Product/1 -> Divide/1
  Hydrogen Molar Mass/1 -> Product2/1
  Number Of Cells/1 -> Product2/2
  Product2/1 -> Divide/2
  Divide/1 -> Current (A)/1
  Hydrogen Flow Rate (kg/s)/1 -> Product/1

== system Final_System_Model_V2/180KW Fuel Cell Stack/Fuel Cell Model/From Pressures (atm) To Nernest Voltage (V)/From Absolute Pressure (atm) To Partial Pressures (atm) ==
  Current Density (i ) : Inport
  Hydrogen Pressure (P_H2) : Inport  Port=2
  Air Pressure (P_air) : Inport  Port=3
  Temperature/C : Inport  Port=4
  Bus Creator : BusCreator  Inputs=5
  Bus Selector : BusSelector  OutputSignals=Air Pressure (atm),Stack Temperature (C),Current Density (A/cm^2),Water Pressure(atm)
  Bus Selector1 : BusSelector  OutputSignals=Stack Temperature (C)
  Bus Selector2 : BusSelector  OutputSignals=Hydrogen Pressure (atm),Stack Temperature (C),Current Density (A/cm^2),Water Pressure(atm)
  Hydrogen Partial Pressure Output : Subsystem
  Oxygen Partial Pressure Output : Subsystem
  Water Pressure output : Subsystem
  Hydrogen Partial Pressure (pp_H2) : Outport
  Oxygen Partial Pressure pp_O2 : Outport  Port=2
  Water Pressure : Outport  Port=3
  wires:
  Water Pressure output/1(Water Pressure) -> Water Pressure/1, Bus Creator/3
  Air Pressure (P_air)/1 -> Bus Creator/1
  Oxygen Partial Pressure Output/1(Oxygen Partial Pressure pp_O2) -> Oxygen Partial Pressure pp_O2/1
  Hydrogen Partial Pressure Output/1(Hydrogen Partial Pressure (pp_H2)) -> Hydrogen Partial Pressure (pp_H2)/1
  Current Density (i )/1 -> Bus Creator/2  "Current Density (A/cm^2)"
  Temperature/C/1 -> Bus Creator/4
  Hydrogen Pressure (P_H2)/1 -> Bus Creator/5
  Bus Creator/1 -> Bus Selector2/1, Bus Selector/1, Bus Selector1/1
  Bus Selector/1 -> Oxygen Partial Pressure Output/1(Air Pressure (P_air))  "<Air Pressure (atm)>"
  Bus Selector/2 -> Oxygen Partial Pressure Output/2(Temperature/C)  "<Stack Temperature (C)>"
  Bus Selector/3 -> Oxygen Partial Pressure Output/3(Current Density/i)  "<Current Density (A/cm^2)>"
  Bus Selector/4 -> Oxygen Partial Pressure Output/4(Water Pressure)  "<Water Pressure(atm)>"
  Bus Selector1/1 -> Water Pressure output/1(Temperature/C)  "<Stack Temperature (C)>"
  Bus Selector2/1 -> Hydrogen Partial Pressure Output/1(Hydrogen Pressure (P_H2))  "<Hydrogen Pressure (atm)>"
  Bus Selector2/2 -> Hydrogen Partial Pressure Output/2(Temperature/C)  "<Stack Temperature (C)>"
  Bus Selector2/3 -> Hydrogen Partial Pressure Output/3(Current Density (i ))  "<Current Density (A/cm^2)>"
  Bus Selector2/4 -> Hydrogen Partial Pressure Output/4(Water Pressure)  "<Water Pressure(atm)>"
